simulink library "libAbcDqFixpt"  (R2013b)
settings: Solver=ode45  StartTime=0.0  StopTime=10.0  RelTol=1e-3
values from neighbouring files (symbols this model uses):
  ctrlConst = struct    [applicationData.m]
libraries: simulink x2, libDataType x1
settings Model: Creator=mcorless  LastModifiedBy=rchladny

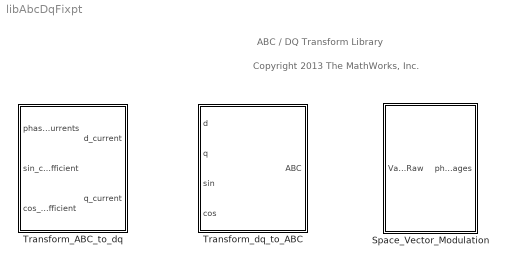
== system libAbcDqFixpt ==
  note: ABC / DQ Transform Library
  note: Copyright 2013 The MathWorks, Inc.
  Space_Vector_Modulation : Subsystem  VariantControl=SpaceVectorModulation_JB
      mask Display: fprintf('SVM')
  Transform_ABC_to_dq : Subsystem  TreatAsAtomicUnit=on  RTWFcnName=TransformABCToDQ
      settings: RTWFcnNameOpts=User specified
      mask Display: disp('Transform\nCoordinates\nABC to dq')
  Transform_dq_to_ABC : Subsystem  TreatAsAtomicUnit=on  RTWFcnName=TransformDQToABCWithSVM
      settings: RTWFcnNameOpts=User specified
      mask Display: disp('Transform\nCoordinates\ndq to ABC')

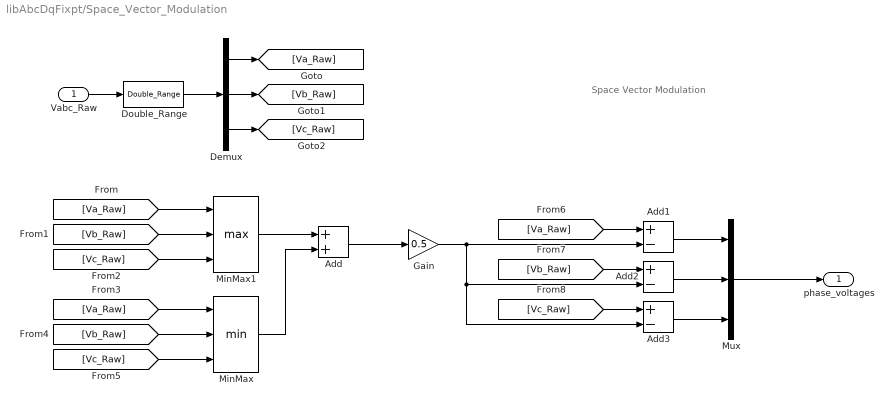
== system libAbcDqFixpt/Space_Vector_Modulation ==
  note: Space Vector Modulation
  Vabc_Raw : Inport
  Add : Sum
  Add1 : Sum  Inputs=+-
  Add2 : Sum  Inputs=+-
  Add3 : Sum  Inputs=+-
  Demux : Demux  Outputs=3
  Double_Range : libDataType/Double_Range  SystemSampleTime=-1
  Gain : Gain  Gain=0.5  OutDataTypeStr=Inherit: Same as input
  MinMax : MinMax  Inputs=3
  MinMax1 : MinMax  Function=max  Inputs=3
  Mux : Mux  Inputs=3
  phase_voltages : Outport
  wires:
  Double_Range/1 -> Demux/1
  Vabc_Raw/1 -> Double_Range/1
  Mux/1 -> phase_voltages/1
  Gain/1 -> Add1/2, Add2/2, Add3/2
  MinMax/1 -> Add/2
  MinMax1/1 -> Add/1
  Add3/1 -> Mux/3
  Add2/1 -> Mux/2
  Add1/1 -> Mux/1
  [Vc_Raw] -> Add3/1
  [Vb_Raw] -> Add2/1
  [Va_Raw] -> Add1/1
  Add/1 -> Gain/1
  [Vc_Raw] -> MinMax/3
  [Vb_Raw] -> MinMax/2
  [Va_Raw] -> MinMax/1
  [Vc_Raw] -> MinMax1/3
  [Vb_Raw] -> MinMax1/2
  [Va_Raw] -> MinMax1/1
  Demux/3 -> [Vc_Raw]
  Demux/2 -> [Vb_Raw]
  Demux/1 -> [Va_Raw]

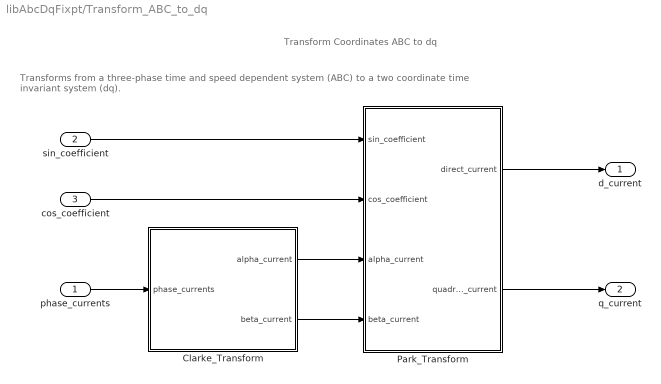
== system libAbcDqFixpt/Transform_ABC_to_dq ==
  note: Transform Coordinates ABC to dq
  note: Transforms from a three-phase time and speed dependent system (ABC) to a two coordinate time invariant system (dq).
  phase_currents : Inport
  sin_coefficient : Inport  Port=2  OutMin=-1  OutMax=1
  cos_coefficient : Inport  Port=3  OutMin=-1  OutMax=1
  Clarke_Transform : Subsystem
  Park_Transform : Subsystem
  d_current : Outport
  q_current : Outport  Port=2
  wires:
  cos_coefficient/1 -> Park_Transform/2(cos_coefficient)
  sin_coefficient/1 -> Park_Transform/1(sin_coefficient)
  phase_currents/1 -> Clarke_Transform/1(phase_currents)
  Park_Transform/2(quadrature_current) -> q_current/1
  Clarke_Transform/1(alpha_current) -> Park_Transform/3(alpha_current)
  Clarke_Transform/2(beta_current) -> Park_Transform/4(beta_current)
  Park_Transform/1(direct_current) -> d_current/1

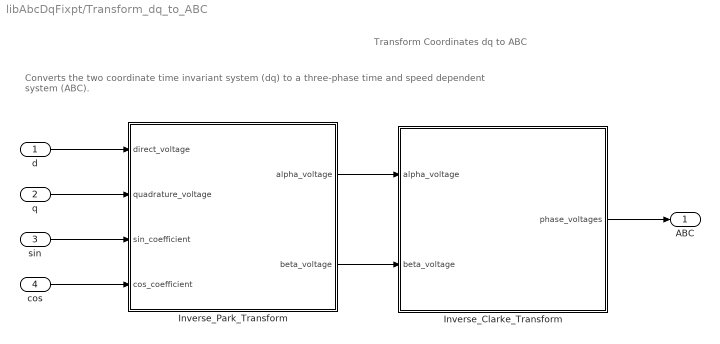
== system libAbcDqFixpt/Transform_dq_to_ABC ==
  note: Transform Coordinates dq to ABC
  note: Converts the two coordinate time invariant system (dq) to a three-phase time and speed dependent system (ABC).
  d : Inport
  q : Inport  Port=2
  sin : Inport  Port=3  OutMin=-1  OutMax=1
  cos : Inport  Port=4  OutMin=-1  OutMax=1
  Inverse_Clarke_Transform : Subsystem  VariantControl=INVERSE_CLARKE_TRANSFORM
  Inverse_Park_Transform : Subsystem
  ABC : Outport
  wires:
  d/1 -> Inverse_Park_Transform/1(direct_voltage)
  Inverse_Park_Transform/1(alpha_voltage) -> Inverse_Clarke_Transform/1(alpha_voltage)
  Inverse_Park_Transform/2(beta_voltage) -> Inverse_Clarke_Transform/2(beta_voltage)
  Inverse_Clarke_Transform/1(phase_voltages) -> ABC/1
  q/1 -> Inverse_Park_Transform/2(quadrature_voltage)
  cos/1 -> Inverse_Park_Transform/4(cos_coefficient)
  sin/1 -> Inverse_Park_Transform/3(sin_coefficient)

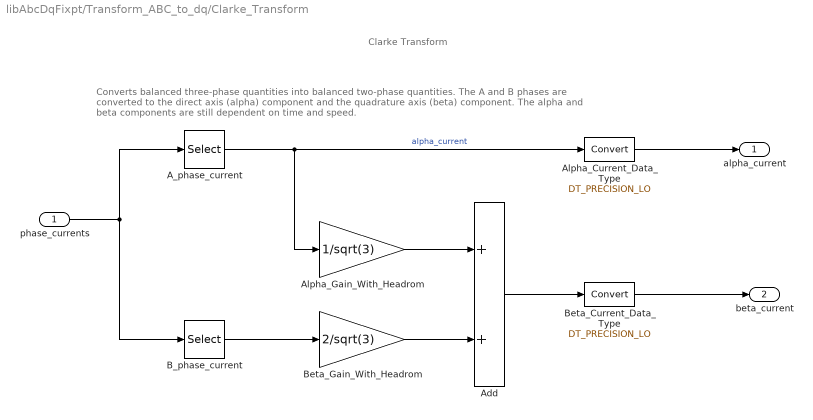
== system libAbcDqFixpt/Transform_ABC_to_dq/Clarke_Transform ==
  note: Clarke Transform
  note: Converts balanced three-phase quantities into balanced two-phase quantities.
      | The A and B phases are converted to the direct axis (alpha) component and the quadrature axis (beta) component.
      | The alpha and beta components are still dependent on time and speed.
  phase_currents : Inport
  A_phase_current : Selector  IndexMode=Zero-based  InputPortWidth=2  IndexOptions=Index vector (dialog)  Indices=0  OutputSizes=1
  Add : Sum  InputSameDT=on  OutDataTypeStr=Inherit: Same as first input
  Alpha_Current_Data_Type : DataTypeConversion  OutMin=-ctrlConst.CurrentMax * 4  OutMax=ctrlConst.CurrentMax * 4  OutDataTypeStr=DT_PRECISION_LO
      settings: AttributesFormatString=--------------------------------------\nMin = %<OutMin>\nMax = %<OutMax>
  Alpha_Gain_With_Headrom : Gain  Gain=1/sqrt(3)  ParamMin=0  ParamMax=(1/sqrt(3)) + (2/sqrt(3))  ParamDataTypeStr=DT_PRECISION_LO
  B_phase_current : Selector  IndexMode=Zero-based  InputPortWidth=2  IndexOptions=Index vector (dialog)  Indices=1  OutputSizes=1
  Beta_Current_Data_Type : DataTypeConversion  OutMin=-ctrlConst.CurrentMax * 4  OutMax=ctrlConst.CurrentMax * 4  OutDataTypeStr=DT_PRECISION_LO
      settings: AttributesFormatString=--------------------------------------\nMin = %<OutMin>\nMax = %<OutMax>
  Beta_Gain_With_Headrom : Gain  Gain=2/sqrt(3)  ParamMin=0  ParamMax=(1/sqrt(3)) + (2/sqrt(3))  ParamDataTypeStr=DT_PRECISION_LO
  alpha_current : Outport
  beta_current : Outport  Port=2
  wires:
  Alpha_Current_Data_Type/1 -> alpha_current/1
  Beta_Current_Data_Type/1 -> beta_current/1
  B_phase_current/1 -> Beta_Gain_With_Headrom/1
  Beta_Gain_With_Headrom/1 -> Add/2
  phase_currents/1 -> A_phase_current/1, B_phase_current/1
  Alpha_Gain_With_Headrom/1 -> Add/1
  A_phase_current/1 -> Alpha_Current_Data_Type/1, Alpha_Gain_With_Headrom/1  "alpha_current"
  Add/1 -> Beta_Current_Data_Type/1

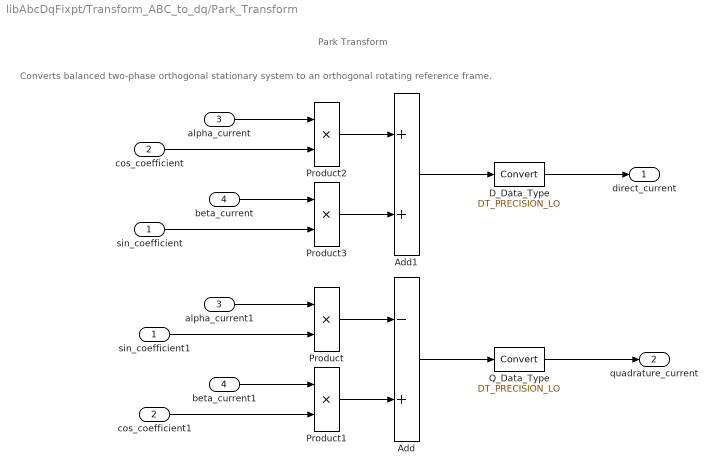
== system libAbcDqFixpt/Transform_ABC_to_dq/Park_Transform ==
  note: Park Transform
  note: Converts balanced two-phase orthogonal stationary system to an orthogonal rotating reference frame.
  sin_coefficient : Inport
  cos_coefficient : Inport  Port=2
  alpha_current : Inport  Port=3
  beta_current : Inport  Port=4
  Add : Sum  Inputs=-+  InputSameDT=on  OutDataTypeStr=Inherit: Same as first input
  Add1 : Sum  InputSameDT=on  OutDataTypeStr=Inherit: Same as first input
  D_Data_Type : DataTypeConversion  OutMin=-ctrlConst.CurrentMax  OutMax=ctrlConst.CurrentMax  OutDataTypeStr=DT_PRECISION_LO  SaturateOnIntegerOverflow=on
      settings: AttributesFormatString=--------------------------------------\nSaturate = %<SaturateOnIntegerOverflow>\nMin = %<OutMin>\nMax = %<OutMax>
  Product{,1..3} (4 alike) : Product  RndMeth=Simplest
  Q_Data_Type : DataTypeConversion  OutMin=-ctrlConst.CurrentMax  OutMax=ctrlConst.CurrentMax  OutDataTypeStr=DT_PRECISION_LO  SaturateOnIntegerOverflow=on
      settings: AttributesFormatString=--------------------------------------\nSaturate = %<SaturateOnIntegerOverflow>\nMin = %<OutMin>\nMax = %<OutMax>
  alpha_current1 : InportShadow  Port=3
  beta_current1 : InportShadow  Port=4
  cos_coefficient1 : InportShadow  Port=2
  sin_coefficient1 : InportShadow
  direct_current : Outport
  quadrature_current : Outport  Port=2
  wires:
  Product/1 -> Add/1
  Product1/1 -> Add/2
  Add/1 -> Q_Data_Type/1
  Product2/1 -> Add1/1
  Product3/1 -> Add1/2
  Add1/1 -> D_Data_Type/1
  alpha_current1/1 -> Product/1
  sin_coefficient1/1 -> Product/2
  cos_coefficient1/1 -> Product1/2
  beta_current1/1 -> Product1/1
  alpha_current/1 -> Product2/1
  cos_coefficient/1 -> Product2/2
  beta_current/1 -> Product3/1
  sin_coefficient/1 -> Product3/2
  D_Data_Type/1 -> direct_current/1
  Q_Data_Type/1 -> quadrature_current/1

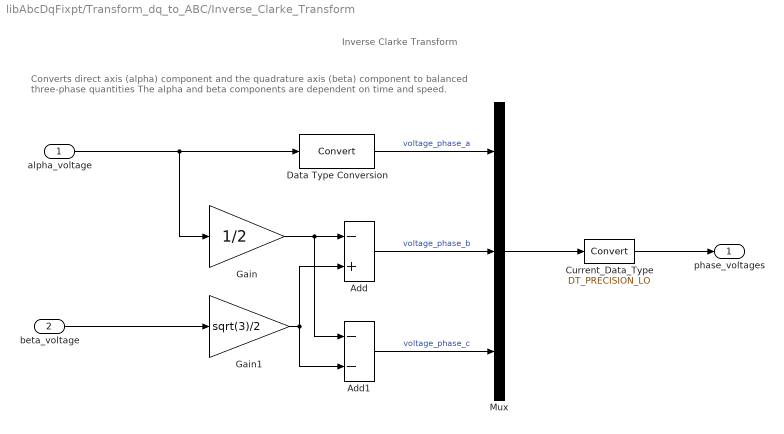
== system libAbcDqFixpt/Transform_dq_to_ABC/Inverse_Clarke_Transform ==
  note: Inverse Clarke Transform
  note: Converts direct axis (alpha) component and the quadrature axis (beta) component to balanced three-phase quantities
      | The alpha and beta components are dependent on time and speed.
  alpha_voltage : Inport
  beta_voltage : Inport  Port=2
  Add : Sum  Inputs=-+  OutDataTypeStr=Inherit: Same as first input
  Add1 : Sum  Inputs=--  OutDataTypeStr=Inherit: Same as first input
  Current_Data_Type : DataTypeConversion  OutMin=-ctrlConst.VoltageMax / 2  OutMax=ctrlConst.VoltageMax /2  OutDataTypeStr=DT_PRECISION_LO  SaturateOnIntegerOverflow=on
      settings: AttributesFormatString=--------------------------------------\nSaturate = %<SaturateOnIntegerOverflow>\nMin = %<OutMin>\nMax = %<OutMax>
  Data Type Conversion : DataTypeConversion
  Gain : Gain  Gain=1/2  ParamMax=1/2 + sqrt(3)/2  ParamDataTypeStr=DT_PRECISION_LO
  Gain1 : Gain  Gain=sqrt(3)/2  ParamMax=1/2 + sqrt(3)/2  ParamDataTypeStr=DT_PRECISION_LO
  Mux : Mux  Inputs=3
  phase_voltages : Outport
  wires:
  Mux/1 -> Current_Data_Type/1
  Gain/1 -> Add1/1, Add/1
  Gain1/1 -> Add1/2, Add/2
  Add/1 -> Mux/2  "voltage_phase_b"
  Add1/1 -> Mux/3  "voltage_phase_c"
  beta_voltage/1 -> Gain1/1
  alpha_voltage/1 -> Gain/1, Data Type Conversion/1
  Data Type Conversion/1 -> Mux/1  "voltage_phase_a"
  Current_Data_Type/1 -> phase_voltages/1

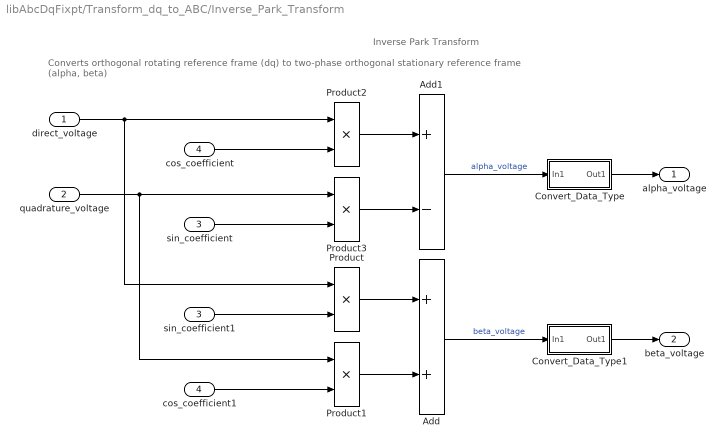
== system libAbcDqFixpt/Transform_dq_to_ABC/Inverse_Park_Transform ==
  note: Inverse Park Transform
  note: Converts orthogonal rotating reference frame (dq) to two-phase orthogonal stationary reference frame (alpha, beta)
  direct_voltage : Inport
  quadrature_voltage : Inport  Port=2
  sin_coefficient : Inport  Port=3
  cos_coefficient : Inport  Port=4
  Add : Sum  InputSameDT=on  OutDataTypeStr=Inherit: Same as first input
  Add1 : Sum  Inputs=+-  InputSameDT=on  OutDataTypeStr=Inherit: Same as first input
  Convert_Data_Type : Subsystem
      mask Display: fprintf('Maintain\nRange')
  Convert_Data_Type1 : Subsystem
      mask Display: fprintf('Maintain\nRange')
  Product{,1..3} (4 alike) : Product  RndMeth=Simplest
  cos_coefficient1 : InportShadow  Port=4
  sin_coefficient1 : InportShadow  Port=3
  alpha_voltage : Outport
  beta_voltage : Outport  Port=2
  wires:
  Convert_Data_Type1/1(Out1) -> beta_voltage/1
  Add/1 -> Convert_Data_Type1/1(In1)  "beta_voltage"
  Convert_Data_Type/1(Out1) -> alpha_voltage/1
  Add1/1 -> Convert_Data_Type/1(In1)  "alpha_voltage"
  Product/1 -> Add/1
  Product1/1 -> Add/2
  Product2/1 -> Add1/1
  Product3/1 -> Add1/2
  cos_coefficient1/1 -> Product1/2
  sin_coefficient/1 -> Product3/2
  direct_voltage/1 -> Product2/1, Product/1
  quadrature_voltage/1 -> Product3/1, Product1/1
  sin_coefficient1/1 -> Product/2
  cos_coefficient/1 -> Product2/2

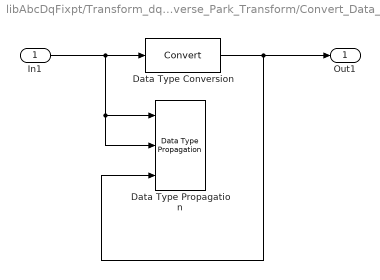
== system libAbcDqFixpt/Transform_dq_to_ABC/Inverse_Park_Transform/Convert_Data_Type ==
  In1 : Inport
  Data Type Conversion : DataTypeConversion
  Data Type Propagation : simulink/Signal Attributes/Data Type Propagation  PropDataTypeMode=Specify via dialog  PropDataType=DT_PRECISION_LO  IfRefDouble=double  IfRefSingle=single  IsSigned=IsSigned1  NumBitsBase=NumBits1  NumBitsMult=0  NumBitsAdd=0  NumBitsAllowFinal=1:128  PropScaling=2^-10  ValuesUsedBestPrec=[5 -7]  SlopeBase=PosRange1  SlopeMult=1  SlopeAdd=0  BiasBase=Bias1  BiasMult=1  BiasAdd=0
      settings: AttributesFormatString=-------------------------------\nDT = %<PropDataType>
  Out1 : Outport
  wires:
  In1/1 -> Data Type Propagation/2, Data Type Propagation/1, Data Type Conversion/1
  Data Type Conversion/1 -> Out1/1, Data Type Propagation/3

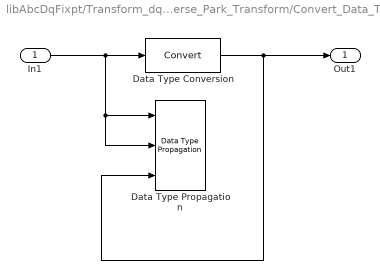
== system libAbcDqFixpt/Transform_dq_to_ABC/Inverse_Park_Transform/Convert_Data_Type1 ==
  In1 : Inport
  Data Type Conversion : DataTypeConversion
  Data Type Propagation : simulink/Signal Attributes/Data Type Propagation  PropDataTypeMode=Specify via dialog  PropDataType=DT_PRECISION_LO  IfRefDouble=double  IfRefSingle=single  IsSigned=IsSigned1  NumBitsBase=NumBits1  NumBitsMult=0  NumBitsAdd=0  NumBitsAllowFinal=1:128  PropScaling=2^-10  ValuesUsedBestPrec=[5 -7]  SlopeBase=PosRange1  SlopeMult=1  SlopeAdd=0  BiasBase=Bias1  BiasMult=1  BiasAdd=0
      settings: AttributesFormatString=-------------------------------\nDT = %<PropDataType>
  Out1 : Outport
  wires:
  In1/1 -> Data Type Propagation/2, Data Type Propagation/1, Data Type Conversion/1
  Data Type Conversion/1 -> Out1/1, Data Type Propagation/3
